simulink model "Final_IHA_2706_2015a"  (R2016b)
settings: Solver=ode5  StartTime=0.0  StopTime=20  FixedStep=SampleTime  RelTol=1e-3  EnableMultiTasking=on
values from neighbouring files (symbols this model uses):
  K = 2000    [code_final.m]
  PowerOn = 0    [code_final.m]
  q = 41.3    [code_final.m]
  Q_AT_break = [-1 -0.7 -0.5 -0.3 -0.2 -0.1 0 0.2 0.8 1]    [code_final.m]
  Q_AT_look = [1 0.1991 0.1227 0.07575 0.04002 0.01761 0.00075 5.86e-8 5.86e-8 5.86e-8]    [code_final.m]
  Q_BT_break = [-1 -0.6 -0.2 0 0.1 0.2 0.3 0.4 0.5 1]    [code_final.m]
  Q_BT_look = [5.86e-8 5.86e-8 5.86e-8 0.000913 0.02175 0.040 0.081 0.10 0.20 1]    [code_final.m]
  Q_PA_break = [-1 -0.6 -0.2 0 0.1 0.2 0.3 0.4 0.5 1]    [code_final.m]
  Q_PA_look = [5.86e-8 5.86e-8 5.86e-8 0.000876 0.0214 0.044 0.071 0.1 0.15 1]    [code_final.m]
  Q_PB_break = [-1 -0.7 -0.5 -0.3 -0.2 -0.1 0 0.2 0.8 1]    [code_final.m]
  Q_PB_look = [1 0.1498 0.1 0.077 0.03591 0.021 0.00082 5.86e-8 5.86e-8 5.86e-8]    [code_final.m]
  SampleTime = .001    (= 0.001)    [code_final.m]
undefined symbols (not defined in the file or in its folder): b, Cylinder, Cylinder1, Cylinder2, Cylinder3, Cylinder4, DiscIntNeverNeededParam, FC, FL1, FL2, FS, Lift, Pillar, Pinion, Piston, Rack, tilt, Valve, VS, X, X1, X2, Y, Z
undefined symbols (not defined in the file): Cyl, HoseA, HoseB, Valve2, Valve3, Valve4
libraries: sm_lib x67, simulink x32, nesl_utility x20, simulink_extras x3, xpcrtudplib x2, xpcobsoletelib x2
(part 1 of 4)
settings Model: Creator=led  LastModifiedBy=led
settings SolverCC: EnableConcurrentExecution=on
settings DataIOCC: SaveFormat=StructureWithTime
settings OptimizationCC: BlockReduction=off  OptimizeBlockIOStorage=off  BufferReuse=off  GlobalBufferReuse=off  ExpressionFolding=off  LocalBlockOutputs=off  LifeSpan=inf
settings DebuggingCC: ReadBeforeWriteMsg=DisableAll  WriteAfterWriteMsg=DisableAll  WriteAfterReadMsg=DisableAll  MultiTaskDSMMsg=none  SFUnexpectedBacktrackingDiag=warning  SFNoUnconditionalDefaultTransitionDiag=warning  SFExecutionAtInitializationDiag=none
settings HardwareCC: ProdBitPerPointer=32  ProdBitPerSizeT=32  ProdBitPerPtrDiffT=32  ProdLargestAtomicFloat=None  ProdWordSize=32  ProdLongLongMode=on  ProdHWDeviceType=Generic->32-bit x86 compatible  TargetBitPerLong=64  TargetBitPerPointer=64  TargetIntDivRoundTo=Zero  TargetEndianess=LittleEndian  TargetWordSize=64  TargetHWDeviceType=Intel->x86-64
settings ModelReferenceCC: UpdateModelReferenceTargets=IfOutOfDate
settings SFSimCC: SFSimEcho=off
settings RTWCC: SystemTargetFile=slrt.tlc  TemplateMakefile=slrt_default_tmf  Description=Simulink Real-Time  RTWCompilerOptimization=on
settings CodeAppCC: MaxIdLength=95
settings SimulinkRealTimeCC: GeneratePreprocessorConditionals=Disable all  xPCisDownloadable=off  xPCisModelTimeout=off  xPCModelTimeoutSecs=20
settings ConfigComp: CovMetricSettings=dw  CovHtmlReporting=on  CovSaveCumulativeToWorkspaceVar=on  CovSaveSingleToWorkspaceVar=on  CovExternalEMLEnable=off

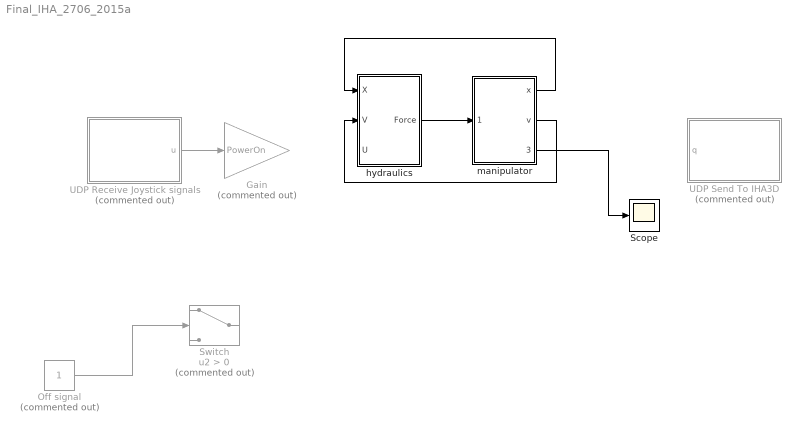
== system Final_IHA_2706_2015a ==
  Gain : Gain  Commented=on  Gain=PowerOn
  Off signal : Constant  Commented=on
  Scope : Scope
  Switch : Switch  Commented=on  Criteria=u2 > Threshold
  UDP Receive Joystick signals : Subsystem  Commented=on
  UDP Send To IHA3D : Subsystem  Commented=on
  hydraulics : Subsystem
  manipulator : Subsystem
  wires:
  manipulator/3(angle joints) -> Scope/1
  manipulator/2(v) -> hydraulics/2(V)
  manipulator/1(x) -> hydraulics/1(X)
  hydraulics/1(Force) -> manipulator/1(Force)
  Off signal/1 -> Switch/2
  UDP Receive Joystick signals/1(u) -> Gain/1

== system Final_IHA_2706_2015a/UDP Receive Joystick signals ==
  Mux : Mux
  Receive signals from Joytick : xpcrtudplib/Legacy UDP/Receive   ipAddress=192.168.10.1  ipPort=55550  width=32  vblLen=off  sampletime=SampleTime
  Terminator : Terminator
  Unpack : xpcobsoletelib/Utilities/Unpack   dimensions={[1],[1],[1],[1]}  datatypes={'double','double','double','double'}  byteAlign=1
  u : Outport
  wires:
  Receive signals from Joytick/2 -> Terminator/1
  Receive signals from Joytick/1 -> Unpack/1
  Unpack/1 -> Mux/1
  Unpack/2 -> Mux/2
  Unpack/3 -> Mux/3
  Unpack/4 -> Mux/4
  Mux/1 -> u/1

== system Final_IHA_2706_2015a/UDP Send To IHA3D ==
  note: Frequency rate:
      | How often UDP message is sent
      | 1: every sample time
      | 2: every second sample time
      | 3: every third sample time
      | 4: etc....
  q : Inport
  Enabled Subsystem : Subsystem  TreatAsAtomicUnit=on
  Frequency rate : Constant  Value=5
  Subsystem : Subsystem
  wires:
  Subsystem/1(enable) -> Enabled Subsystem/Enable
  Frequency rate/1 -> Subsystem/1(freq)
  q/1 -> Enabled Subsystem/1(q)

== system Final_IHA_2706_2015a/hydraulics ==
  X : Inport
  V : Inport  Port=2
  U : Inport  Port=3
  Cylinder1 : Subsystem
  Cylinder2 : Subsystem
  Cylinder3 : Subsystem
  Cylinder4 : Subsystem
  Demux3 : Demux
  Demux4 : Demux
  Demux5 : Demux
  Mux1 : Mux
  Mux2 : Mux
  Sine Wave{,1..3} (4 alike) : Sin  SineType=Sample based  Amplitude=0.5  Samples=10000  SampleTime=SampleTime
  Force : Outport
  wires:
  Demux5/2 -> Cylinder2/1(Cylinder2_x)
  Demux4/2 -> Cylinder2/2(Cylinder2_v)
  Mux2/1 -> Force/1
  X/1 -> Demux5/1
  Demux5/1 -> Cylinder1/1(Cylinder1_x)
  V/1 -> Demux4/1
  Demux4/1 -> Cylinder1/2(Cylinder1_v)
  Demux5/3 -> Cylinder3/1(Cylinder3_x)
  Demux4/3 -> Cylinder3/2(Cylinder3_v)
  Demux4/4 -> Cylinder4/2(Cylinder4_v)
  Demux5/4 -> Cylinder4/1(Cylinder4_x)
  Cylinder4/1(Cylinder4_Force) -> Mux2/4
  Cylinder1/1(Cylinder1_Force) -> Mux2/1
  Cylinder2/1(Cylinder2_Force) -> Mux2/2
  Cylinder3/1(Cylinder3_Force) -> Mux2/3
  Demux3/1 -> Cylinder1/3(Uvalve)
  Demux3/2 -> Cylinder2/3(Uvalve)
  Demux3/3 -> Cylinder3/3(Uvalve)
  Demux3/4 -> Cylinder4/3(Uvalve)
  Sine Wave/1 -> Mux1/1
  Sine Wave2/1 -> Mux1/3
  Sine Wave3/1 -> Mux1/4
  Sine Wave1/1 -> Mux1/2
  Mux1/1 -> Demux3/1

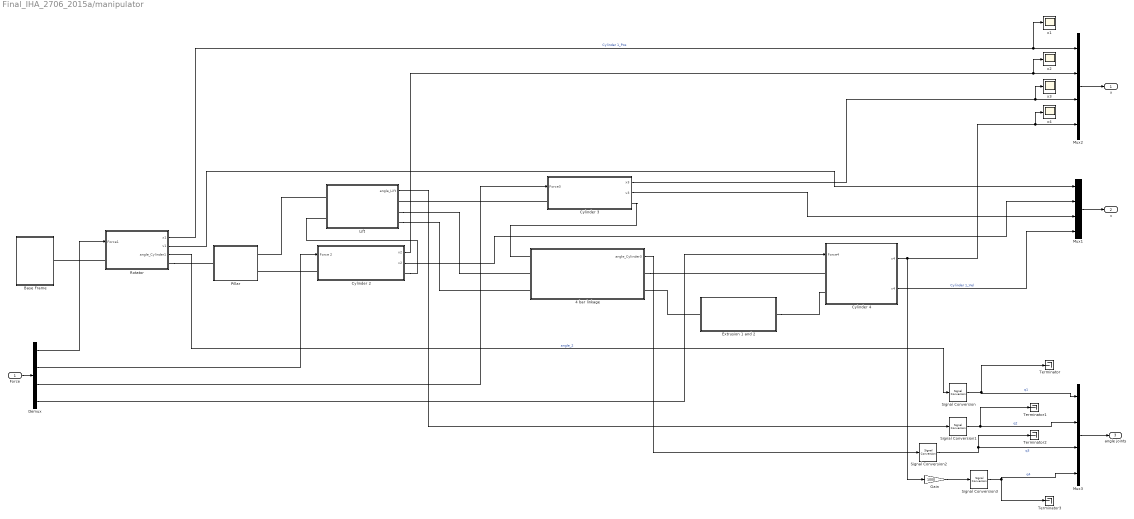
== system Final_IHA_2706_2015a/manipulator ==
  Force : Inport
  4 bar linkage : Subsystem
  Base Frame : Subsystem
  Cylinder 2 : Subsystem
  Cylinder 3 : Subsystem
  Cylinder 4 : Subsystem
  Demux : Demux
  Extrusion 1 and 2 : Subsystem
  Gain : Gain  Gain=1000
  Lift : Subsystem
  Mux1 : Mux
  Mux2 : Mux
  Mux3 : Mux
  Pillar : Subsystem
  Rotator : Subsystem
  Signal Conversion{,1..3} (4 alike) : SignalConversion  OverrideOpt=off
  Terminator{,1..3} (4 alike) : Terminator
  x{1..4} (4 alike) : Scope
  x : Outport
  v : Outport  Port=2
  angle joints : Outport  Port=3
  wires:
  Mux2/1 -> x/1
  Mux1/1 -> v/1
  Mux3/1 -> angle joints/1
  Force/1 -> Demux/1
  Gain/1 -> Signal Conversion3/1
  Signal Conversion/1 -> Mux3/1, Terminator/1  "q1"
  Signal Conversion1/1 -> Terminator1/1, Mux3/2  "q2"
  Signal Conversion2/1 -> Terminator2/1, Mux3/3  "q3"
  Signal Conversion3/1 -> Mux3/4, Terminator3/1  "q4"
  Demux/1 -> Rotator/1(Force1)
  Demux/2 -> Cylinder 2/1(Force 2)
  Demux/3 -> Cylinder 3/1(Force3)
  Demux/4 -> Cylinder 4/1(Force4)
  Cylinder 4/1(x4) -> Gain/1, x4/1, Mux2/4
  Cylinder 4/2(v4) -> Mux1/4  "Cylinder 1_Vel"
  Cylinder 3/2(v3) -> Mux1/3
  Cylinder 2/2(v2) -> Mux1/2
  Cylinder 2/1(x2) -> x2/1, Mux2/2
  Rotator/2(v1) -> Mux1/1
  Rotator/1(x1) -> x1/1, Mux2/1  "Cylinder 1_Pos"
  Rotator/3(angle_Cylinder1) -> Signal Conversion/1  "angle_2"
  Lift/1(angle_Lift) -> Signal Conversion1/1
  4 bar linkage/1(angle_Cylinder3) -> Signal Conversion2/1
  Cylinder 3/1(x3) -> x3/1, Mux2/3
  connections:
  Extrusion 1 and 2/RConn1 -- Cylinder 4/LConn2
  Rotator/LConn1 -- Base Frame/RConn1
  Rotator/RConn1 -- Pillar/LConn1
  Cylinder 2/LConn1 -- Pillar/RConn2
  Cylinder 2/RConn1 -- Lift/LConn2
  Lift/LConn1 -- Pillar/RConn1
  Cylinder 3/LConn1 -- Lift/RConn1
  Cylinder 3/RConn1 -- 4 bar linkage/LConn1
  Lift/RConn2 -- 4 bar linkage/LConn2
  Lift/RConn3 -- 4 bar linkage/LConn3
  Extrusion 1 and 2/LConn1 -- 4 bar linkage/RConn2
  4 bar linkage/RConn1 -- Cylinder 4/LConn1

== system Final_IHA_2706_2015a/UDP Send To IHA3D/Enabled Subsystem ==
  q : Inport
  Enable : EnablePort
  Add : Sum  Inputs=--
  Demux : Demux
  Pack1 : xpcobsoletelib/Utilities/Pack   datatypes={'uint8','double','double','double','double','double','double'}  byteAlign=1
  Send1 : xpcrtudplib/Legacy UDP/Send   ipAddress=192.168.10.1  ipPort=7755  localPort=5555  vblLen=off  sampletime=SampleTime
  UDP header : Constant  Value=[0 0 0 0 0 1 0 8]  OutDataTypeStr=uint8
  wires:
  UDP header/1 -> Pack1/1  "header"
  q/1 -> Demux/1
  Demux/2 -> Pack1/3, Add/1  "lift"
  Demux/3 -> Pack1/4, Add/2  "tilt"
  Demux/4 -> Pack1/6, Pack1/5  "ext"
  Add/1 -> Pack1/7  "grap"
  Demux/1 -> Pack1/2  "turn"
  Pack1/1 -> Send1/1

== system Final_IHA_2706_2015a/UDP Send To IHA3D/Subsystem ==
  freq : Inport
  Digital Clock : DigitalClock  SampleTime=SampleTime
  Fcn1 : Fcn  Expr=(u(1)<=0.001)*1
  Gain : Gain  Gain=1000
  Gain1 : Gain  Gain=1000
  Math Function : Math  Operator=mod  SaturateOnIntegerOverflow=on
  Weighted Sample Time : SampleTimeMath  TsampMathOp=*
  enable : Outport
  wires:
  Weighted Sample Time/1 -> Math Function/2
  freq/1 -> Gain1/1
  Math Function/1 -> Fcn1/1
  Gain/1 -> Math Function/1
  Gain1/1 -> Weighted Sample Time/1
  Fcn1/1 -> enable/1
  Digital Clock/1 -> Gain/1

== system Final_IHA_2706_2015a/hydraulics/Cylinder1 ==
  Cylinder1_x : Inport
  Cylinder1_v : Inport  Port=2
  Uvalve : Inport  Port=3
  Add1 : Sum  Inputs=++-
  Constant : Constant
  Cylinder1 : Subsystem  mask(Hydraulic){D=[Cylinder.D Cylinder.r1/2], xmax=Cylinder1.max, Vdead=[1e-4  1e-4], Vhose=[0 0], B_o=Cyl.BulkMod, Bhose=[HoseA.Bulk HoseB.Bulk], pini=[Cylinder1.pA   Valve.SupplyP]}
      mask prompts: D "Diameters of piston and piston rod [m  m] :"; xmax "Cylindes stroke [m] :"; Vdead "Dead volumes at cylinder ends [m^3  m^3] :"; Vhose "Volumes of hoses [m^3  m^3] :"; B_o "Bulk modulus of oil [Pa] :"; Bhose "Bulk moduli of hoses [Pa  Pa] :"; pini "Initial pressures [Pa Pa] :"
      mask init:
      | A_A = pi/4*D(1)^2; A_B = A_A-pi/4*D(2)^2; V_0A = Vdead(1); V_0B = Vdead(2); V_HA = Vhose(1); V_HB = Vhose(2); B_HA = Bhose(1); B_HB = Bhose(2); p_0A = pini(1); p_0B = pini(2);
  Demux : Demux  Outputs=2
  Endforce_model : Subsystem
  Friction_model : Subsystem
  Gain : Gain  Commented=through  Gain=PowerOn
  Gain1 : Gain  Gain=Valve.SupplyP
  Mux : Mux  Inputs=2
  Tank Pressure : Constant  Value=0
  Valve System1 : Subsystem
  Cylinder1_Force : Outport
  wires:
  Demux/2 -> Valve System1/3(p_B)
  Mux/1 -> Cylinder1/1(QA & QB)
  Valve System1/2(Q_B) -> Mux/2
  Cylinder1/1(pA & pB) -> Demux/1
  Demux/1 -> Valve System1/1(p_A)
  Valve System1/1(Q_A) -> Mux/1
  Tank Pressure/1 -> Valve System1/5(p_T)
  Uvalve/1 -> Valve System1/2(Uvalve)
  Cylinder1_v/1 -> Endforce_model/2(v), Cylinder1/3(dx/dt), Friction_model/1(v1)
  Cylinder1_x/1 -> Endforce_model/1(x), Cylinder1/2(x)
  Cylinder1/2(F) -> Add1/1
  Add1/1 -> Cylinder1_Force/1
  Endforce_model/1(F_end) -> Add1/2
  Friction_model/1(Friction_Force_1) -> Add1/3
  Gain/1 -> Valve System1/4(p_S)
  Gain1/1 -> Gain/1
  Constant/1 -> Gain1/1

== system Final_IHA_2706_2015a/hydraulics/Cylinder2 ==
  Cylinder2_x : Inport
  Cylinder2_v : Inport  Port=2
  Uvalve : Inport  Port=3
  Add1 : Sum  Inputs=++-
  Cylinder2 : Subsystem  mask(Hydraulic){D=[Cylinder2.D Cylinder.r2/2], xmax=Cylinder2.max, Vdead=[1e-4  1e-4], Vhose=[0 0], B_o=Cyl.BulkMod, Bhose=[HoseA.Bulk HoseB.Bulk], pini=[Cylinder2.pA   Valve.SupplyP]}
      mask prompts: D "Diameters of piston and piston rod [m  m] :"; xmax "Cylindes stroke [m] :"; Vdead "Dead volumes at cylinder ends [m^3  m^3] :"; Vhose "Volumes of hoses [m^3  m^3] :"; B_o "Bulk modulus of oil [Pa] :"; Bhose "Bulk moduli of hoses [Pa  Pa] :"; pini "Initial pressures [Pa Pa] :"
      mask init:
      | A_A = pi/4*D(1)^2; A_B = A_A-pi/4*D(2)^2; V_0A = Vdead(1); V_0B = Vdead(2); V_HA = Vhose(1); V_HB = Vhose(2); B_HA = Bhose(1); B_HB = Bhose(2); p_0A = pini(1); p_0B = pini(2);
  Demux : Demux  Outputs=2
  Endforce_model : Subsystem
  Friction_model : Subsystem
  Gain : Gain  Commented=through  Gain=PowerOn
  Mux : Mux  Inputs=2
  Supply Pressure : Constant  Value=Valve.SupplyP
  Tank Pressure : Constant  Value=0
  Valve System2 : Subsystem
  Cylinder2_Force : Outport
  wires:
  Supply Pressure/1 -> Gain/1
  Friction_model/1(Friction_Force) -> Add1/3
  Endforce_model/1(End_Force) -> Add1/2
  Add1/1 -> Cylinder2_Force/1
  Cylinder2/2(F) -> Add1/1
  Cylinder2_x/1 -> Cylinder2/2(x), Endforce_model/1(x)
  Cylinder2_v/1 -> Friction_model/1(v), Cylinder2/3(dx/dt), Endforce_model/2(v)
  Uvalve/1 -> Valve System2/2(Uvalve)
  Tank Pressure/1 -> Valve System2/5(p_T)
  Valve System2/1(Q_A) -> Mux/1
  Demux/1 -> Valve System2/1(p_A)
  Cylinder2/1(pA & pB) -> Demux/1
  Valve System2/2(Q_B) -> Mux/2
  Mux/1 -> Cylinder2/1(QA & QB)
  Demux/2 -> Valve System2/3(p_B)
  Gain/1 -> Valve System2/4(p_S)

== system Final_IHA_2706_2015a/hydraulics/Cylinder3 ==
  Cylinder3_x : Inport
  Cylinder3_v : Inport  Port=2
  Uvalve : Inport  Port=3
  Add1 : Sum  Inputs=++-
  Cylinder3 : Subsystem  mask(Hydraulic){D=[Cylinder3.D Cylinder.r3/2], xmax=Cylinder3.max, Vdead=[1e-4  1e-4], Vhose=[0 0], B_o=Cyl.BulkMod, Bhose=[HoseA.Bulk HoseB.Bulk], pini=[Cylinder3.pA   Valve.SupplyP]}
      mask prompts: D "Diameters of piston and piston rod [m  m] :"; xmax "Cylindes stroke [m] :"; Vdead "Dead volumes at cylinder ends [m^3  m^3] :"; Vhose "Volumes of hoses [m^3  m^3] :"; B_o "Bulk modulus of oil [Pa] :"; Bhose "Bulk moduli of hoses [Pa  Pa] :"; pini "Initial pressures [Pa Pa] :"
      mask init:
      | A_A = pi/4*D(1)^2; A_B = A_A-pi/4*D(2)^2; V_0A = Vdead(1); V_0B = Vdead(2); V_HA = Vhose(1); V_HB = Vhose(2); B_HA = Bhose(1); B_HB = Bhose(2); p_0A = pini(1); p_0B = pini(2);
  Demux : Demux  Outputs=2
  Endforce_model : Subsystem
  Friction_model : Subsystem
  Gain : Gain  Commented=through  Gain=PowerOn
  Mux : Mux  Inputs=2
  Supply Pressure : Constant  Value=Valve.SupplyP
  Tank Pressure : Constant  Value=0
  Valve System3 : Subsystem
  Cylinder3_Force : Outport
  wires:
  Demux/2 -> Valve System3/3(p_B)
  Mux/1 -> Cylinder3/1(QA & QB)
  Valve System3/2(Q_B) -> Mux/2
  Cylinder3/1(pA & pB) -> Demux/1
  Demux/1 -> Valve System3/1(p_A)
  Valve System3/1(Q_A) -> Mux/1
  Tank Pressure/1 -> Valve System3/5(p_T)
  Uvalve/1 -> Valve System3/2(Uvalve)
  Cylinder3_v/1 -> Endforce_model/2(v), Cylinder3/3(dx/dt), Friction_model/1(v)
  Cylinder3_x/1 -> Endforce_model/1(x), Cylinder3/2(x)
  Cylinder3/2(F) -> Add1/1
  Add1/1 -> Cylinder3_Force/1
  Endforce_model/1(End_Force) -> Add1/2
  Friction_model/1(Friction_Force) -> Add1/3
  Supply Pressure/1 -> Gain/1
  Gain/1 -> Valve System3/4(p_S)

== system Final_IHA_2706_2015a/hydraulics/Cylinder4 ==
  Cylinder4_x : Inport
  Cylinder4_v : Inport  Port=2
  Uvalve : Inport  Port=3
  Add1 : Sum  Inputs=++-
  Cylinder4 : Subsystem  mask(Hydraulic){D=[Cylinder4.D Cylinder.r4/2], xmax=Cylinder4.max, Vdead=[1e-4  1e-4], Vhose=[0 0], B_o=Cyl.BulkMod, Bhose=[HoseA.Bulk HoseB.Bulk], pini=[Cylinder4.pA   Valve.SupplyP]}
      mask prompts: D "Diameters of piston and piston rod [m  m] :"; xmax "Cylindes stroke [m] :"; Vdead "Dead volumes at cylinder ends [m^3  m^3] :"; Vhose "Volumes of hoses [m^3  m^3] :"; B_o "Bulk modulus of oil [Pa] :"; Bhose "Bulk moduli of hoses [Pa  Pa] :"; pini "Initial pressures [Pa Pa] :"
      mask init:
      | A_A = pi/4*D(1)^2; A_B = A_A-pi/4*D(2)^2; V_0A = Vdead(1); V_0B = Vdead(2); V_HA = Vhose(1); V_HB = Vhose(2); B_HA = Bhose(1); B_HB = Bhose(2); p_0A = pini(1); p_0B = pini(2);
  Demux : Demux  Outputs=2
  Endforce_model : Subsystem
  Friction_model : Subsystem
  Gain : Gain  Commented=through  Gain=PowerOn
  Mux : Mux  Inputs=2
  Supply Pressure : Constant  Value=Valve.SupplyP
  Tank Pressure : Constant  Value=0
  Valve System4 : Subsystem
  Cylinder4_Force : Outport
  wires:
  Supply Pressure/1 -> Gain/1
  Friction_model/1(Friction_Force) -> Add1/3
  Endforce_model/1(End_Force) -> Add1/2
  Add1/1 -> Cylinder4_Force/1
  Cylinder4/2(F) -> Add1/1
  Cylinder4_x/1 -> Cylinder4/2(x), Endforce_model/1(x)
  Cylinder4_v/1 -> Friction_model/1(v), Cylinder4/3(dx/dt), Endforce_model/2(v)
  Uvalve/1 -> Valve System4/2(Uvalve)
  Tank Pressure/1 -> Valve System4/5(p_T)
  Valve System4/1(Q_A) -> Mux/1
  Demux/1 -> Valve System4/1(p_A)
  Cylinder4/1(pA & pB) -> Demux/1
  Valve System4/2(Q_B) -> Mux/2
  Mux/1 -> Cylinder4/1(QA & QB)
  Demux/2 -> Valve System4/3(p_B)
  Gain/1 -> Valve System4/4(p_S)

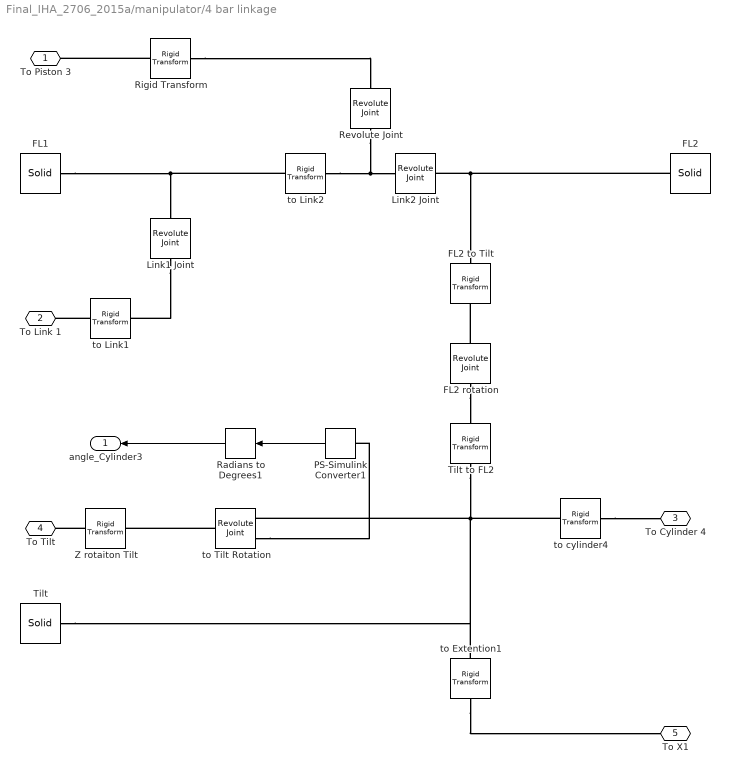
== system Final_IHA_2706_2015a/manipulator/4 bar linkage ==
  FL1 : sm_lib/Body Elements/Solid  InertiaType=Custom  Mass=FL1.m  MassUnits=kg  CenterOfMass=FL1.cm  CenterOfMassUnits=m  MomentsOfInertia=[1 1 1]  MomentsOfInertiaUnits=kg*m^2  ProductsOfInertia=[0 0 0]  ProductsOfInertiaUnits=kg*m^2  DensityBased=on  Density=1000  DensityUnits=kg/(m^3)  DoExposeReferenceFrame=on  SerializedFrames=<Frames/>  GraphicType=FromGeometry  MarkerShape=Sphere  MarkerSize=10  MarkerSizeUnits=m  GraphicVisPropType=SimpleVisualProperties  GraphicDiffuseColor=FL1.rgb  GraphicSpecularColor=[0.5 0.5 0.5 1.0]  GraphicAmbientColor=[0.15 0.15 0.15 1.0]  GraphicEmissiveColor=[0.0 0.0 0.0 1.0]  GraphicShininess=75  GraphicOpacity=1.0  GeometryShape=GeneralExtrusion  RectangleSize=[1 1]  RectangleSizeUnits=m  BrickDimensions=[1 1 1]  BrickDimensionUnits=m  CylinderRadius=1  CylinderRadiusUnits=m  CylinderLength=1  CylinderLengthUnits=m  SphereRadius=1  SphereRadiusUnits=m  EllipsoidRadii=[1 1 1]  EllipsoidRadiiUnits=m  ExtrusionCrossSection=FL1.c  ExtrusionCrossSectionUnits=m  ExtrusionLength=FL1.l  ExtrusionLengthUnits=m  PolygonNumSides=3  PolygonOuterRadius=1  PolygonOuterRadiusUnits=m  ExtGeomFileType=STEP  ExtGeomFileUnits=m  RevolutionCrossSection=[1 1; 1 -1; 2 -1; 2 1]  RevolutionCrossSectionUnits=m  RevolutionExtent=Full  RevolutionAngle=180  RevolutionAngleUnits=deg
  FL2 : sm_lib/Body Elements/Solid  InertiaType=Custom  Mass=FL2.m  MassUnits=kg  CenterOfMass=FL2.cm  CenterOfMassUnits=m  MomentsOfInertia=[1 1 1]  MomentsOfInertiaUnits=kg*m^2  ProductsOfInertia=[0 0 0]  ProductsOfInertiaUnits=kg*m^2  DensityBased=on  Density=1000  DensityUnits=kg/(m^3)  DoExposeReferenceFrame=on  SerializedFrames=<Frames/>  GraphicType=FromGeometry  MarkerShape=Sphere  MarkerSize=10  MarkerSizeUnits=m  GraphicVisPropType=SimpleVisualProperties  GraphicDiffuseColor=FL2.rgb  GraphicSpecularColor=[0.5 0.5 0.5 1.0]  GraphicAmbientColor=[0.15 0.15 0.15 1.0]  GraphicEmissiveColor=[0.0 0.0 0.0 1.0]  GraphicShininess=75  GraphicOpacity=1.0  GeometryShape=GeneralExtrusion  RectangleSize=[1 1]  RectangleSizeUnits=m  BrickDimensions=[1 1 1]  BrickDimensionUnits=m  CylinderRadius=1  CylinderRadiusUnits=m  CylinderLength=1  CylinderLengthUnits=m  SphereRadius=1  SphereRadiusUnits=m  EllipsoidRadii=[1 1 1]  EllipsoidRadiiUnits=m  ExtrusionCrossSection=FL2.c  ExtrusionCrossSectionUnits=m  ExtrusionLength=FL2.l  ExtrusionLengthUnits=m  PolygonNumSides=3  PolygonOuterRadius=1  PolygonOuterRadiusUnits=m  ExtGeomFileType=STEP  ExtGeomFileUnits=m  RevolutionCrossSection=[1 1; 1 -1; 2 -1; 2 1]  RevolutionCrossSectionUnits=m  RevolutionExtent=Full  RevolutionAngle=180  RevolutionAngleUnits=deg
  FL2 rotation : sm_lib/Joints/Revolute Joint  SenseConstraintForce=off  SenseConstraintForceX=off  SenseConstraintForceY=off  SenseConstraintForceZ=off  SenseConstraintTorque=off  SenseConstraintTorqueX=off  SenseConstraintTorqueY=off  SenseConstraintTorqueZ=off  SenseTotalForce=off  SenseTotalForceX=off  SenseTotalForceY=off  SenseTotalForceZ=off  SenseTotalTorque=off  SenseTotalTorqueX=off  SenseTotalTorqueY=off  SenseTotalTorqueZ=off  CompositeWrenchDir=FollowerOnBase  CompositeWrenchFrame=BaseFrame  EquilibriumPosition=0  EquilibriumPositionUnits=deg  SpringStiffness=0  SpringStiffnessUnits=N*m/deg  DampingCoefficient=0  DampingCoefficientUnits=N*m/(deg/s)  TorqueActuationMode=NoTorque  MotionActuationMode=ComputedMotion  SensePosition=off  SenseVelocity=off  SenseAcceleration=off  SenseTorqueForce=off  PositionTargetSpecify=off  PositionTargetPriority=High  PositionTargetValue=0  PositionTargetValueUnits=deg  VelocityTargetSpecify=off  VelocityTargetPriority=High  VelocityTargetValue=0  VelocityTargetValueUnits=deg/s
  FL2 to Tilt : sm_lib/Frames and Transforms/Rigid Transform  TranslationMethod=Cartesian  TranslationStandardOffset=0  TranslationLengthUnit=m  TranslationStandardAxis=+Z  TranslationCartesianOffset=FL2pos.j  TranslationROffset=0  TranslationROffsetUnits=m  TranslationZOffset=0  TranslationZOffsetUnits=m  TranslationThetaOffset=0  TranslationThetaOffsetUnits=deg  RotationMethod=None  RotationAngleUnits=deg  RotationStandardAxis=+Z  RotationAngle=0.0  RotationArbitraryAxis=[0 0 1]  FollAlignAxisA=+X  BaseAlignAxisA=+Y  FollAlignAxisB=+Y  BaseAlignAxisB=+Z  RotationSequenceAxes=FollowerAxes  RotationSequence=XYX  RotationSequenceAngles=[0 0 0]  RotationSequenceAnglesUnits=deg  RotationMatrix=[1 0 0; 0 1 0; 0 0 1]
  Link1 Joint : sm_lib/Joints/Revolute Joint  SenseConstraintForce=off  SenseConstraintForceX=off  SenseConstraintForceY=off  SenseConstraintForceZ=off  SenseConstraintTorque=off  SenseConstraintTorqueX=off  SenseConstraintTorqueY=off  SenseConstraintTorqueZ=off  SenseTotalForce=off  SenseTotalForceX=off  SenseTotalForceY=off  SenseTotalForceZ=off  SenseTotalTorque=off  SenseTotalTorqueX=off  SenseTotalTorqueY=off  SenseTotalTorqueZ=off  CompositeWrenchDir=FollowerOnBase  CompositeWrenchFrame=BaseFrame  EquilibriumPosition=0  EquilibriumPositionUnits=deg  SpringStiffness=0  SpringStiffnessUnits=N*m/deg  DampingCoefficient=0  DampingCoefficientUnits=N*m/(deg/s)  TorqueActuationMode=NoTorque  MotionActuationMode=ComputedMotion  SensePosition=off  SenseVelocity=off  SenseAcceleration=off  SenseTorqueForce=off  PositionTargetSpecify=on  PositionTargetPriority=Low  PositionTargetValue=90  PositionTargetValueUnits=deg  VelocityTargetSpecify=off  VelocityTargetPriority=High  VelocityTargetValue=0  VelocityTargetValueUnits=deg/s
  Link2 Joint : sm_lib/Joints/Revolute Joint  SenseConstraintForce=off  SenseConstraintForceX=off  SenseConstraintForceY=off  SenseConstraintForceZ=off  SenseConstraintTorque=off  SenseConstraintTorqueX=off  SenseConstraintTorqueY=off  SenseConstraintTorqueZ=off  SenseTotalForce=off  SenseTotalForceX=off  SenseTotalForceY=off  SenseTotalForceZ=off  SenseTotalTorque=off  SenseTotalTorqueX=off  SenseTotalTorqueY=off  SenseTotalTorqueZ=off  CompositeWrenchDir=FollowerOnBase  CompositeWrenchFrame=BaseFrame  EquilibriumPosition=0  EquilibriumPositionUnits=deg  SpringStiffness=0  SpringStiffnessUnits=N*m/deg  DampingCoefficient=0  DampingCoefficientUnits=N*m/(deg/s)  TorqueActuationMode=NoTorque  MotionActuationMode=ComputedMotion  SensePosition=off  SenseVelocity=off  SenseAcceleration=off  SenseTorqueForce=off  PositionTargetSpecify=on  PositionTargetPriority=Low  PositionTargetValue=0  PositionTargetValueUnits=deg  VelocityTargetSpecify=off  VelocityTargetPriority=High  VelocityTargetValue=0  VelocityTargetValueUnits=deg/s
  PS-Simulink Converter1 : nesl_utility/PS-Simulink Converter  PhysicalDomain=network_engine_domain  SubClassName=ps_output  LeftPortType=input  RightPortType=output  PseudoPeriodic=off  Frequencies=[]  Unit=1  AffineConversion=off
  Radians to Degrees1 : simulink_extras/Transformations/Radians to Degrees
  Revolute Joint : sm_lib/Joints/Revolute Joint  SenseConstraintForce=off  SenseConstraintForceX=off  SenseConstraintForceY=off  SenseConstraintForceZ=off  SenseConstraintTorque=off  SenseConstraintTorqueX=off  SenseConstraintTorqueY=off  SenseConstraintTorqueZ=off  SenseTotalForce=off  SenseTotalForceX=off  SenseTotalForceY=off  SenseTotalForceZ=off  SenseTotalTorque=off  SenseTotalTorqueX=off  SenseTotalTorqueY=off  SenseTotalTorqueZ=off  CompositeWrenchDir=FollowerOnBase  CompositeWrenchFrame=BaseFrame  EquilibriumPosition=0  EquilibriumPositionUnits=deg  SpringStiffness=0  SpringStiffnessUnits=N*m/deg  DampingCoefficient=0  DampingCoefficientUnits=N*m/(deg/s)  TorqueActuationMode=NoTorque  MotionActuationMode=ComputedMotion  SensePosition=off  SenseVelocity=off  SenseAcceleration=off  SenseTorqueForce=off  PositionTargetSpecify=off  PositionTargetPriority=High  PositionTargetValue=0  PositionTargetValueUnits=deg  VelocityTargetSpecify=off  VelocityTargetPriority=High  VelocityTargetValue=0  VelocityTargetValueUnits=deg/s
  Rigid Transform : sm_lib/Frames and Transforms/Rigid Transform  TranslationMethod=StandardAxis  TranslationStandardOffset=Piston.l3/2  TranslationLengthUnit=m  TranslationStandardAxis=-X  TranslationCartesianOffset=[0 0 0]  TranslationROffset=0  TranslationROffsetUnits=m  TranslationZOffset=0  TranslationZOffsetUnits=m  TranslationThetaOffset=0  TranslationThetaOffsetUnits=deg  RotationMethod=StandardAxis  RotationAngleUnits=deg  RotationStandardAxis=+Y  RotationAngle=90  RotationArbitraryAxis=[0 0 1]  FollAlignAxisA=+X  BaseAlignAxisA=+Y  FollAlignAxisB=+Y  BaseAlignAxisB=+Z  RotationSequenceAxes=FollowerAxes  RotationSequence=XYX  RotationSequenceAngles=[0 0 0]  RotationSequenceAnglesUnits=deg  RotationMatrix=[1 0 0; 0 1 0; 0 0 1]
  Tilt : sm_lib/Body Elements/Solid  InertiaType=Custom  Mass=tilt.m  MassUnits=kg  CenterOfMass=tilt.cm  CenterOfMassUnits=m  MomentsOfInertia=[1 1 1]  MomentsOfInertiaUnits=kg*m^2  ProductsOfInertia=[0 0 0]  ProductsOfInertiaUnits=kg*m^2  DensityBased=on  Density=1000  DensityUnits=kg/(m^3)  DoExposeReferenceFrame=on  SerializedFrames=<Frames/>  GraphicType=FromGeometry  MarkerShape=Sphere  MarkerSize=10  MarkerSizeUnits=m  GraphicVisPropType=SimpleVisualProperties  GraphicDiffuseColor=tilt.rgb  GraphicSpecularColor=[0.5 0.5 0.5 1.0]  GraphicAmbientColor=[0.15 0.15 0.15 1.0]  GraphicEmissiveColor=[0.0 0.0 0.0 1.0]  GraphicShininess=75  GraphicOpacity=1.0  GeometryShape=GeneralExtrusion  RectangleSize=[1 1]  RectangleSizeUnits=m  BrickDimensions=[1 1 1]  BrickDimensionUnits=m  CylinderRadius=1  CylinderRadiusUnits=m  CylinderLength=1  CylinderLengthUnits=m  SphereRadius=1  SphereRadiusUnits=m  EllipsoidRadii=[1 1 1]  EllipsoidRadiiUnits=m  ExtrusionCrossSection=tilt.c  ExtrusionCrossSectionUnits=m  ExtrusionLength=tilt.l  ExtrusionLengthUnits=m  PolygonNumSides=3  PolygonOuterRadius=1  PolygonOuterRadiusUnits=m  ExtGeomFileType=STEP  ExtGeomFileUnits=m  RevolutionCrossSection=[1 1; 1 -1; 2 -1; 2 1]  RevolutionCrossSectionUnits=m  RevolutionExtent=Full  RevolutionAngle=180  RevolutionAngleUnits=deg
  Tilt to FL2 : sm_lib/Frames and Transforms/Rigid Transform  TranslationMethod=Cartesian  TranslationStandardOffset=0  TranslationLengthUnit=m  TranslationStandardAxis=+Z  TranslationCartesianOffset=tiltpos.j  TranslationROffset=0  TranslationROffsetUnits=m  TranslationZOffset=0  TranslationZOffsetUnits=m  TranslationThetaOffset=0  TranslationThetaOffsetUnits=deg  RotationMethod=None  RotationAngleUnits=deg  RotationStandardAxis=+Z  RotationAngle=0.0  RotationArbitraryAxis=[0 0 1]  FollAlignAxisA=+X  BaseAlignAxisA=+Y  FollAlignAxisB=+Y  BaseAlignAxisB=+Z  RotationSequenceAxes=FollowerAxes  RotationSequence=XYX  RotationSequenceAngles=[0 0 0]  RotationSequenceAnglesUnits=deg  RotationMatrix=[1 0 0; 0 1 0; 0 0 1]
  Z rotaiton Tilt : sm_lib/Frames and Transforms/Rigid Transform  TranslationMethod=Cartesian  TranslationStandardOffset=0  TranslationLengthUnit=m  TranslationStandardAxis=+Z  TranslationCartesianOffset=tilt.j  TranslationROffset=0  TranslationROffsetUnits=m  TranslationZOffset=0  TranslationZOffsetUnits=m  TranslationThetaOffset=0  TranslationThetaOffsetUnits=deg  RotationMethod=None  RotationAngleUnits=deg  RotationStandardAxis=+Z  RotationAngle=0.0  RotationArbitraryAxis=[0 0 1]  FollAlignAxisA=+X  BaseAlignAxisA=+Y  FollAlignAxisB=+Y  BaseAlignAxisB=+Z  RotationSequenceAxes=FollowerAxes  RotationSequence=XYX  RotationSequenceAngles=[0 0 0]  RotationSequenceAnglesUnits=deg  RotationMatrix=[1 0 0; 0 1 0; 0 0 1]
  to Extention1 : sm_lib/Frames and Transforms/Rigid Transform  TranslationMethod=Cartesian  TranslationStandardOffset=0  TranslationLengthUnit=m  TranslationStandardAxis=+Z  TranslationCartesianOffset=X1.pos  TranslationROffset=0  TranslationROffsetUnits=m  TranslationZOffset=0  TranslationZOffsetUnits=m  TranslationThetaOffset=0  TranslationThetaOffsetUnits=deg  RotationMethod=StandardAxis  RotationAngleUnits=deg  RotationStandardAxis=+Y  RotationAngle=90  RotationArbitraryAxis=[0 0 1]  FollAlignAxisA=+X  BaseAlignAxisA=+Y  FollAlignAxisB=+Y  BaseAlignAxisB=+Z  RotationSequenceAxes=FollowerAxes  RotationSequence=XYX  RotationSequenceAngles=[0 0 0]  RotationSequenceAnglesUnits=deg  RotationMatrix=[1 0 0; 0 1 0; 0 0 1]
  to Link1 : sm_lib/Frames and Transforms/Rigid Transform  TranslationMethod=Cartesian  TranslationStandardOffset=0  TranslationLengthUnit=m  TranslationStandardAxis=+Z  TranslationCartesianOffset=FL1.j  TranslationROffset=0  TranslationROffsetUnits=m  TranslationZOffset=0  TranslationZOffsetUnits=m  TranslationThetaOffset=0  TranslationThetaOffsetUnits=deg  RotationMethod=None  RotationAngleUnits=deg  RotationStandardAxis=+Z  RotationAngle=0.0  RotationArbitraryAxis=[0 0 1]  FollAlignAxisA=+X  BaseAlignAxisA=+Y  FollAlignAxisB=+Y  BaseAlignAxisB=+Z  RotationSequenceAxes=FollowerAxes  RotationSequence=XYX  RotationSequenceAngles=[0 0 0]  RotationSequenceAnglesUnits=deg  RotationMatrix=[1 0 0; 0 1 0; 0 0 1]
  to Link2 : sm_lib/Frames and Transforms/Rigid Transform  TranslationMethod=Cartesian  TranslationStandardOffset=0  TranslationLengthUnit=m  TranslationStandardAxis=+Z  TranslationCartesianOffset=FL2.j  TranslationROffset=0  TranslationROffsetUnits=m  TranslationZOffset=0  TranslationZOffsetUnits=m  TranslationThetaOffset=0  TranslationThetaOffsetUnits=deg  RotationMethod=None  RotationAngleUnits=deg  RotationStandardAxis=+Z  RotationAngle=0.0  RotationArbitraryAxis=[0 0 1]  FollAlignAxisA=+X  BaseAlignAxisA=+Y  FollAlignAxisB=+Y  BaseAlignAxisB=+Z  RotationSequenceAxes=FollowerAxes  RotationSequence=XYX  RotationSequenceAngles=[0 0 0]  RotationSequenceAnglesUnits=deg  RotationMatrix=[1 0 0; 0 1 0; 0 0 1]
  to Tilt Rotation : sm_lib/Joints/Revolute Joint  SenseConstraintForce=off  SenseConstraintForceX=off  SenseConstraintForceY=off  SenseConstraintForceZ=off  SenseConstraintTorque=off  SenseConstraintTorqueX=off  SenseConstraintTorqueY=off  SenseConstraintTorqueZ=off  SenseTotalForce=off  SenseTotalForceX=off  SenseTotalForceY=off  SenseTotalForceZ=off  SenseTotalTorque=off  SenseTotalTorqueX=off  SenseTotalTorqueY=off  SenseTotalTorqueZ=off  CompositeWrenchDir=FollowerOnBase  CompositeWrenchFrame=BaseFrame  EquilibriumPosition=0  EquilibriumPositionUnits=deg  SpringStiffness=0  SpringStiffnessUnits=N*m/deg  DampingCoefficient=0  DampingCoefficientUnits=N*m/(deg/s)  TorqueActuationMode=NoTorque  MotionActuationMode=ComputedMotion  SensePosition=on  SenseVelocity=off  SenseAcceleration=off  SenseTorqueForce=off  PositionTargetSpecify=off  PositionTargetPriority=Low  PositionTargetValue=90  PositionTargetValueUnits=deg  VelocityTargetSpecify=off  VelocityTargetPriority=High  VelocityTargetValue=0  VelocityTargetValueUnits=deg/s
  to cylinder4 : sm_lib/Frames and Transforms/Rigid Transform  TranslationMethod=Cartesian  TranslationStandardOffset=0  TranslationLengthUnit=m  TranslationStandardAxis=+Z  TranslationCartesianOffset=Cylinder.pos4  TranslationROffset=0  TranslationROffsetUnits=m  TranslationZOffset=0  TranslationZOffsetUnits=m  TranslationThetaOffset=0  TranslationThetaOffsetUnits=deg  RotationMethod=None  RotationAngleUnits=deg  RotationStandardAxis=+Z  RotationAngle=0.0  RotationArbitraryAxis=[0 0 1]  FollAlignAxisA=+X  BaseAlignAxisA=+Y  FollAlignAxisB=+Y  BaseAlignAxisB=+Z  RotationSequenceAxes=FollowerAxes  RotationSequence=XYX  RotationSequenceAngles=[0 0 0]  RotationSequenceAnglesUnits=deg  RotationMatrix=[1 0 0; 0 1 0; 0 0 1]
  To Piston 3 : PMIOPort  Port=1  Side=Left
  To Link 1 : PMIOPort  Port=2  Side=Left
  To Cylinder 4 : PMIOPort  Port=3  Side=Right
  To Tilt : PMIOPort  Port=4  Side=Left
  To X1 : PMIOPort  Port=5  Side=Right
  angle_Cylinder3 : Outport
  wires:
  Radians to Degrees1/1 -> angle_Cylinder3/1
  PS-Simulink Converter1/1 -> Radians to Degrees1/1
  connections:
  to cylinder4/RConn1 -- To Cylinder 4/RConn1
  to Link1/LConn1 -- To Link 1/RConn1
  Z rotaiton Tilt/LConn1 -- To Tilt/RConn1
  Rigid Transform/RConn1 -- To Piston 3/RConn1
  to Extention1/RConn1 -- To X1/RConn1
  to cylinder4/LConn1 -- to Tilt Rotation/RConn1 -- Tilt to FL2/LConn1 -- to Extention1/LConn1 -- Tilt/RConn1
  FL2/RConn1 -- Link2 Joint/RConn1 -- FL2 to Tilt/LConn1
  Revolute Joint/LConn1 -- Link2 Joint/LConn1 -- to Link2/RConn1
  FL1/RConn1 -- to Link2/LConn1 -- Link1 Joint/RConn1
  FL2 rotation/LConn1 -- Tilt to FL2/RConn1
  Link1 Joint/LConn1 -- to Link1/RConn1
  Rigid Transform/LConn1 -- Revolute Joint/RConn1
  FL2 rotation/RConn1 -- FL2 to Tilt/RConn1
  to Tilt Rotation/LConn1 -- Z rotaiton Tilt/RConn1
  to Tilt Rotation/RConn2 -- PS-Simulink Converter1/LConn1

== system Final_IHA_2706_2015a/manipulator/Base Frame ==
  Mechanism Configuration : sm_lib/Utilities/Mechanism Configuration  UniformGravity=Constant  GravityVector=[0 -9.81 0]  GravityUnits=m/s^2  LinearizationDelta=0.001
  "Pinion " : sm_lib/Frames and Transforms/Rigid Transform  TranslationMethod=Cartesian  TranslationStandardOffset=0  TranslationLengthUnit=m  TranslationStandardAxis=+Z  TranslationCartesianOffset=Pinion.j/2  TranslationROffset=0  TranslationROffsetUnits=m  TranslationZOffset=0  TranslationZOffsetUnits=m  TranslationThetaOffset=0  TranslationThetaOffsetUnits=deg  RotationMethod=None  RotationAngleUnits=deg  RotationStandardAxis=+Z  RotationAngle=0.0  RotationArbitraryAxis=[0 0 1]  FollAlignAxisA=+X  BaseAlignAxisA=+Y  FollAlignAxisB=+Y  BaseAlignAxisB=+Z  RotationSequenceAxes=FollowerAxes  RotationSequence=XYX  RotationSequenceAngles=[0 0 0]  RotationSequenceAnglesUnits=deg  RotationMatrix=[1 0 0; 0 1 0; 0 0 1]
  Solver Configuration : nesl_utility/Solver Configuration  PhysicalDomain=network_engine_domain  SubClassName=solver  LeftPortType=input  RightPortType=generic  Accelerate=off  Tones=[]  Harmonics=[]  SimulateNoise=off  Profile=off  UseLocalSampling=off  EnableSwitchedLinearOptims=on  FrequencyDomain=off  UseCCode=off  RelTol=0.001  AbsTol=1e-06  MinStep=1e-09  ToWorkspace=off  RevertToSquareIcSolve=off  NumHomotopyIterations=100  PhasorMode=off  PhasorModeNumHarmonics=1  OverrideAbsTol=off  DoDC=off  ResidualTolerance=1e-09  UseLocalSolver=off  LocalSolverChoice=NE_BACKWARD_EULER_ADVANCER  LocalSolverSampleTime=0.001  DoFixedCost=off  MaxNonlinIter=3  MaxModeIter=2  LinearAlgebra=Sparse  DelaysMemoryBudget=1024  AutomaticFiltering=on  FilteringTimeConstant=0.001
  World Frame : sm_lib/Frames and Transforms/World Frame
  to Pinion : sm_lib/Frames and Transforms/Rigid Transform  TranslationMethod=None  TranslationStandardOffset=0  TranslationLengthUnit=m  TranslationStandardAxis=+Z  TranslationCartesianOffset=[0 0 0]  TranslationROffset=0  TranslationROffsetUnits=m  TranslationZOffset=0  TranslationZOffsetUnits=m  TranslationThetaOffset=0  TranslationThetaOffsetUnits=deg  RotationMethod=AlignedAxes  RotationAngleUnits=deg  RotationStandardAxis=+Z  RotationAngle=0.0  RotationArbitraryAxis=[0 0 1]  FollAlignAxisA=+Z  BaseAlignAxisA=+Y  FollAlignAxisB=+Y  BaseAlignAxisB=+X  RotationSequenceAxes=FollowerAxes  RotationSequence=XYX  RotationSequenceAngles=[0 0 0]  RotationSequenceAnglesUnits=deg  RotationMatrix=[1 0 0; 0 1 0; 0 0 1]
  Base : PMIOPort  Port=1  Side=Right
  connections:
  Solver Configuration/RConn1 -- Mechanism Configuration/RConn1 -- World Frame/RConn1 -- "Pinion "/LConn1
  to Pinion/RConn1 -- Base/RConn1
  to Pinion/LConn1 -- "Pinion "/RConn1

== system Final_IHA_2706_2015a/manipulator/Cylinder 2 ==
  Force 2 : Inport
  Cylinder 2 : sm_lib/Body Elements/Solid  InertiaType=Custom  Mass=Cylinder.m2  MassUnits=kg  CenterOfMass=Cylinder.cm2  CenterOfMassUnits=m  MomentsOfInertia=[1 1 1]  MomentsOfInertiaUnits=kg*m^2  ProductsOfInertia=[0 0 0]  ProductsOfInertiaUnits=kg*m^2  DensityBased=on  Density=1000  DensityUnits=kg/(m^3)  DoExposeReferenceFrame=on  SerializedFrames=<Frames/>  GraphicType=FromGeometry  MarkerShape=Sphere  MarkerSize=10  MarkerSizeUnits=m  GraphicVisPropType=SimpleVisualProperties  GraphicDiffuseColor=Cylinder.rgb  GraphicSpecularColor=[0.5 0.5 0.5 1.0]  GraphicAmbientColor=[0.15 0.15 0.15 1.0]  GraphicEmissiveColor=[0.0 0.0 0.0 1.0]  GraphicShininess=75  GraphicOpacity=1.0  GeometryShape=Cylinder  RectangleSize=[1 1]  RectangleSizeUnits=m  BrickDimensions=[1 1 1]  BrickDimensionUnits=m  CylinderRadius=Cylinder.r2  CylinderRadiusUnits=m  CylinderLength=Cylinder.l2  CylinderLengthUnits=m  SphereRadius=1  SphereRadiusUnits=m  EllipsoidRadii=[1 1 1]  EllipsoidRadiiUnits=m  ExtrusionCrossSection=Lift.c  ExtrusionCrossSectionUnits=m  ExtrusionLength=Lift.l  ExtrusionLengthUnits=m  PolygonNumSides=3  PolygonOuterRadius=1  PolygonOuterRadiusUnits=m  ExtGeomFileType=STEP  ExtGeomFileUnits=m  RevolutionCrossSection=[1 1; 1 -1; 2 -1; 2 1]  RevolutionCrossSectionUnits=m  RevolutionExtent=Full  RevolutionAngle=180  RevolutionAngleUnits=deg
  Cylinder 2 Joint : sm_lib/Joints/Prismatic Joint  SenseConstraintForce=off  SenseConstraintForceX=off  SenseConstraintForceY=off  SenseConstraintForceZ=off  SenseConstraintTorque=off  SenseConstraintTorqueX=off  SenseConstraintTorqueY=off  SenseConstraintTorqueZ=off  SenseTotalForce=off  SenseTotalForceX=off  SenseTotalForceY=off  SenseTotalForceZ=off  SenseTotalTorque=off  SenseTotalTorqueX=off  SenseTotalTorqueY=off  SenseTotalTorqueZ=off  CompositeWrenchDir=FollowerOnBase  CompositeWrenchFrame=BaseFrame  EquilibriumPosition=0  EquilibriumPositionUnits=m  SpringStiffness=0  SpringStiffnessUnits=N/m  DampingCoefficient=0  DampingCoefficientUnits=N/(m/s)  TorqueActuationMode=InputTorque  MotionActuationMode=ComputedMotion  SensePosition=on  SenseVelocity=on  SenseAcceleration=off  SenseTorqueForce=off  PositionTargetSpecify=off  PositionTargetPriority=High  PositionTargetValue=0  PositionTargetValueUnits=m  VelocityTargetSpecify=off  VelocityTargetPriority=High  VelocityTargetValue=0  VelocityTargetValueUnits=m/s
  Cylinder 2 con : sm_lib/Joints/Revolute Joint  SenseConstraintForce=off  SenseConstraintForceX=off  SenseConstraintForceY=off  SenseConstraintForceZ=off  SenseConstraintTorque=off  SenseConstraintTorqueX=off  SenseConstraintTorqueY=off  SenseConstraintTorqueZ=off  SenseTotalForce=off  SenseTotalForceX=off  SenseTotalForceY=off  SenseTotalForceZ=off  SenseTotalTorque=off  SenseTotalTorqueX=off  SenseTotalTorqueY=off  SenseTotalTorqueZ=off  CompositeWrenchDir=FollowerOnBase  CompositeWrenchFrame=BaseFrame  EquilibriumPosition=0  EquilibriumPositionUnits=deg  SpringStiffness=0  SpringStiffnessUnits=N*m/deg  DampingCoefficient=0  DampingCoefficientUnits=N*m/(deg/s)  TorqueActuationMode=NoTorque  MotionActuationMode=ComputedMotion  SensePosition=off  SenseVelocity=off  SenseAcceleration=off  SenseTorqueForce=off  PositionTargetSpecify=off  PositionTargetPriority=High  PositionTargetValue=0  PositionTargetValueUnits=deg  VelocityTargetSpecify=off  VelocityTargetPriority=High  VelocityTargetValue=0  VelocityTargetValueUnits=deg/s
  PS-Simulink Converter : nesl_utility/PS-Simulink Converter  PhysicalDomain=network_engine_domain  SubClassName=ps_output  LeftPortType=input  RightPortType=output  PseudoPeriodic=off  Frequencies=[]  Unit=1  AffineConversion=off
  PS-Simulink Converter1 : nesl_utility/PS-Simulink Converter  PhysicalDomain=network_engine_domain  SubClassName=ps_output  LeftPortType=input  RightPortType=output  PseudoPeriodic=off  Frequencies=[]  Unit=1  AffineConversion=off
  Piston 2 : sm_lib/Body Elements/Solid  InertiaType=Custom  Mass=Piston.m2  MassUnits=kg  CenterOfMass=Piston.cm2  CenterOfMassUnits=m  MomentsOfInertia=[1 1 1]  MomentsOfInertiaUnits=kg*m^2  ProductsOfInertia=[0 0 0]  ProductsOfInertiaUnits=kg*m^2  DensityBased=on  Density=1000  DensityUnits=kg/(m^3)  DoExposeReferenceFrame=on  SerializedFrames=<Frames/>  GraphicType=FromGeometry  MarkerShape=Sphere  MarkerSize=10  MarkerSizeUnits=m  GraphicVisPropType=SimpleVisualProperties  GraphicDiffuseColor=Piston.rgb  GraphicSpecularColor=[0.5 0.5 0.5 1.0]  GraphicAmbientColor=[0.15 0.15 0.15 1.0]  GraphicEmissiveColor=[0.0 0.0 0.0 1.0]  GraphicShininess=75  GraphicOpacity=1.0  GeometryShape=Cylinder  RectangleSize=[1 1]  RectangleSizeUnits=m  BrickDimensions=[1 1 1]  BrickDimensionUnits=m  CylinderRadius=Piston.r2  CylinderRadiusUnits=m  CylinderLength=Piston.l2  CylinderLengthUnits=m  SphereRadius=1  SphereRadiusUnits=m  EllipsoidRadii=[1 1 1]  EllipsoidRadiiUnits=m  ExtrusionCrossSection=Lift.c  ExtrusionCrossSectionUnits=m  ExtrusionLength=Lift.l  ExtrusionLengthUnits=m  PolygonNumSides=3  PolygonOuterRadius=1  PolygonOuterRadiusUnits=m  ExtGeomFileType=STEP  ExtGeomFileUnits=m  RevolutionCrossSection=[1 1; 1 -1; 2 -1; 2 1]  RevolutionCrossSectionUnits=m  RevolutionExtent=Full  RevolutionAngle=180  RevolutionAngleUnits=deg
  Piston 2 con : sm_lib/Joints/Revolute Joint  SenseConstraintForce=off  SenseConstraintForceX=off  SenseConstraintForceY=off  SenseConstraintForceZ=off  SenseConstraintTorque=off  SenseConstraintTorqueX=off  SenseConstraintTorqueY=off  SenseConstraintTorqueZ=off  SenseTotalForce=off  SenseTotalForceX=off  SenseTotalForceY=off  SenseTotalForceZ=off  SenseTotalTorque=off  SenseTotalTorqueX=off  SenseTotalTorqueY=off  SenseTotalTorqueZ=off  CompositeWrenchDir=FollowerOnBase  CompositeWrenchFrame=BaseFrame  EquilibriumPosition=0  EquilibriumPositionUnits=deg  SpringStiffness=0  SpringStiffnessUnits=N*m/deg  DampingCoefficient=0  DampingCoefficientUnits=N*m/(deg/s)  TorqueActuationMode=NoTorque  MotionActuationMode=ComputedMotion  SensePosition=off  SenseVelocity=off  SenseAcceleration=off  SenseTorqueForce=off  PositionTargetSpecify=off  PositionTargetPriority=High  PositionTargetValue=0  PositionTargetValueUnits=deg  VelocityTargetSpecify=off  VelocityTargetPriority=High  VelocityTargetValue=0  VelocityTargetValueUnits=deg/s
  Simulink-PS Converter : nesl_utility/Simulink-PS Converter  PhysicalDomain=network_engine_domain  SubClassName=ps_input  LeftPortType=input  RightPortType=output  PseudoPeriodic=off  Frequencies=[]  NoiseDistribution=none  NoiseParameters=[]  Unit=1  AffineConversion=off  InputFiltering=off  SimscapeFilterOrder=1  InputFilterTimeConstant=0.001  UdotUserProvided=1
  to Cylinder 2 Solid : sm_lib/Frames and Transforms/Rigid Transform  TranslationMethod=StandardAxis  TranslationStandardOffset=Cylinder.l2/2  TranslationLengthUnit=m  TranslationStandardAxis=-Y  TranslationCartesianOffset=Lift.j  TranslationROffset=0  TranslationROffsetUnits=m  TranslationZOffset=0  TranslationZOffsetUnits=m  TranslationThetaOffset=0  TranslationThetaOffsetUnits=deg  RotationMethod=StandardAxis  RotationAngleUnits=deg  RotationStandardAxis=-X  RotationAngle=90  RotationArbitraryAxis=[0 0 1]  FollAlignAxisA=+X  BaseAlignAxisA=+Y  FollAlignAxisB=+Y  BaseAlignAxisB=+Z  RotationSequenceAxes=FollowerAxes  RotationSequence=XYX  RotationSequenceAngles=[0 0 0]  RotationSequenceAnglesUnits=deg  RotationMatrix=[1 0 0; 0 1 0; 0 0 1]
  to Piston 2 Solid : sm_lib/Frames and Transforms/Rigid Transform  TranslationMethod=StandardAxis  TranslationStandardOffset=Piston.l2/2  TranslationLengthUnit=m  TranslationStandardAxis=+Y  TranslationCartesianOffset=Lift.j  TranslationROffset=0  TranslationROffsetUnits=m  TranslationZOffset=0  TranslationZOffsetUnits=m  TranslationThetaOffset=0  TranslationThetaOffsetUnits=deg  RotationMethod=StandardAxis  RotationAngleUnits=deg  RotationStandardAxis=-X  RotationAngle=90  RotationArbitraryAxis=[0 0 1]  FollAlignAxisA=+X  BaseAlignAxisA=+Y  FollAlignAxisB=+Y  BaseAlignAxisB=+Z  RotationSequenceAxes=FollowerAxes  RotationSequence=XYX  RotationSequenceAngles=[0 0 0]  RotationSequenceAnglesUnits=deg  RotationMatrix=[1 0 0; 0 1 0; 0 0 1]
  ToPillar : PMIOPort  Port=1  Side=Left
  ToLift : PMIOPort  Port=2  Side=Right
  x2 : Outport
  v2 : Outport  Port=2
  wires:
  PS-Simulink Converter/1 -> x2/1
  PS-Simulink Converter1/1 -> v2/1
  Force 2/1 -> Simulink-PS Converter/1
  connections:
  ToPillar/RConn1 -- Piston 2 con/LConn1
  Piston 2 con/RConn1 -- to Piston 2 Solid/LConn1
  to Cylinder 2 Solid/RConn1 -- Cylinder 2/RConn1 -- Cylinder 2 Joint/RConn1
  to Piston 2 Solid/RConn1 -- Piston 2/RConn1 -- Cylinder 2 Joint/LConn1
  ToLift/RConn1 -- Cylinder 2 con/LConn1
  Cylinder 2 con/RConn1 -- to Cylinder 2 Solid/LConn1
  Simulink-PS Converter/RConn1 -- Cylinder 2 Joint/LConn2
  Cylinder 2 Joint/RConn2 -- PS-Simulink Converter/LConn1
  PS-Simulink Converter1/LConn1 -- Cylinder 2 Joint/RConn3
